simulink model "Multi_agent_system"  (R2016b)
settings: Solver=VariableStepAuto  StartTime=0.0  StopTime=10  RelTol=1e-3
values from neighbouring files (symbols this model uses):
  A = [ 0  1  0 ... (first row only)    [config.m]
  a = 1    [config.m]
  b = 1    [config.m]
  c = 1    [config.m]
  n = 3    [config.m]
  v = 1 + 1/r    (= 1.5)    [config.m]
  x_initial = [0 ... (first row only)    [config.m]
settings Model: Creator=kvlton  LastModifiedBy=kvlton

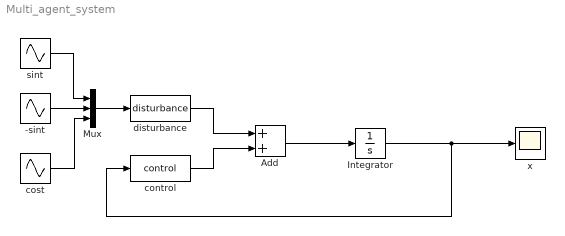
== system Multi_agent_system ==
  -sint : Sin  Amplitude=-1  SampleTime=0
  Add : Sum
  Integrator : Integrator  InitialCondition=x_initial*100
  Mux : Mux  Inputs=3
  control : S-Function  FunctionName=control  Parameters=A,n,a,b,c,u,v  SFunctionDeploymentMode=off  EnableBusSupport=off
  cost : Sin  Phase=pi/2  SampleTime=0
  disturbance : S-Function  FunctionName=disturbance  Parameters=n  SFunctionDeploymentMode=off  EnableBusSupport=off
  sint : Sin  SampleTime=0
  x : Scope
  wires:
  Integrator/1 -> control/1, x/1
  control/1 -> Add/2
  disturbance/1 -> Add/1
  Add/1 -> Integrator/1
  sint/1 -> Mux/1
  -sint/1 -> Mux/2
  cost/1 -> Mux/3
  Mux/1 -> disturbance/1
